simulink library "dspspect2"  (Simulink 3.00)
undefined symbols (not defined in the file or in its folder): magnitude
libraries: dspspect2 x5, dspparest2 x4, dspbdsp2 x2, dspxfrm2 x1, simulink x1, dsparch2 x1
settings Model: Creator=don  LastModifiedBy=surekha

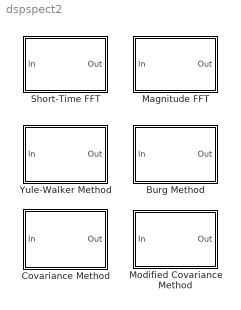
== system dspspect2 ==
  Burg Method : Subsystem  mask(Burg Method){fftsize=256, ord=6}
      mask prompts: fftsize "FFT length (-1 to inherit input width):"; ord "Order:"
      mask help: Frame-based parametric estimation of the AR spectrum using the Burg Method.
      mask init:
      | d = 0.1; xe=4; x=-xe:d:xe;
      | y = ones(size(x)); i=find(x); y(i)=sin(pi*x(i))./(pi*x(i));
      | y = abs(y).^(0.75);
      mask Help: web(dspbhelp);
      mask Display: text(-3,1.2,'Burg'); plot(-xe,0,xe,1.3,x,y)
  Covariance Method : Subsystem  mask(Covariance Method){bufsiz=128, fftsize=256, ord=6}
      mask prompts: bufsiz "Input frame size:"; fftsize "FFT length (-1 to inherit input width):"; ord "Order:"
      mask help: Frame-based parametric estimation of the AR spectrum using the Covariance Method.
      mask init:
      | d = 0.1; xe=4; x=-xe:d:xe;
      | y = ones(size(x)); i=find(x); y(i)=sin(pi*x(i))./(pi*x(i));
      | y = abs(y).^(0.75);
      mask Help: web(dspbhelp);
      mask Display: text(-3,1.2,'Cov AR'); plot(-xe,0,xe,1.3,x,y)
  Magnitude FFT : Subsystem  mask(Magnitude FFT){fftsize=128, NChans=1}
      mask prompts: fftsize "FFT length (-1 to inherit input width):"; NChans "Number of channels:"
      mask help: Compute magnitude-squared FFT of input frame, with optional zero padding.
      mask Help: web(dspbhelp);
      mask Display: disp('|FFT| ^ 2')
  Modified Covariance Method : Subsystem  mask(Modified Covariance Method){bufsiz=128, fftsize=256, ord=6}
      mask prompts: bufsiz "Input frame size:"; fftsize "FFT length (-1 to inherit input width):"; ord "Order:"
      mask help: Frame-based parametric estimation of the AR spectrum using the Modified Covariance Method.
      mask init:
      | d = 0.1; xe=4; x=-xe:d:xe;
      | y = ones(size(x)); i=find(x); y(i)=sin(pi*x(i))./(pi*x(i));
      | y = abs(y).^(0.75);
      mask Help: web(dspbhelp);
      mask Display: text(-3,1.2,'MCov AR'); plot(-xe,0,xe,1.3,x,y)
  Short-Time FFT : Subsystem  mask(Short-Time FFT){fftsize=256, navg=4, wintype=Hamming, Rs=50, beta=5, winsamp=Symmetric, NChans=1}
      mask prompts: fftsize "FFT length (-1 to inherit input width):"; navg "Number of spectral averages:"; wintype "Window type:"; Rs "Stopband attenuation in dB:"; winsamp "Window sampling:"; NChans "Number of channels:"
      mask help: Frame-based nonparametric spectral estimation using the short-time FFT.
      mask init:
      | [x,y,xe]=dspblkperiodogram('icon');
      mask Help: web(dspbhelp);
      mask StyleString: edit,edit,popup(Bartlett|Blackman|Boxcar|Chebyshev|Hamming|Hann|Hanning|Kaiser|Triang),edit,edit,popup(Symmetric|Periodic),edit
      mask CallbackString: ||dspblkperiodogram||||
      mask Display: text(-3,1.15,'ST-FFT'); plot(-xe,0,xe,1.3,x,y)
  Yule-Walker Method : Subsystem  mask(Yule-Walker Method){fftsize=256, ord=6}
      mask prompts: fftsize "FFT length (-1 to inherit input width):"; ord "Order:"
      mask help: Frame-based parametric estimation of the AR spectrum using the autocorrelation (LPC) method.
      mask init:
      | d = 0.1; xe=4; x=-xe:d:xe;
      | y = ones(size(x)); i=find(x); y(i)=sin(pi*x(i))./(pi*x(i));
      | y = abs(y).^(0.75);
      mask Help: web(dspbhelp);
      mask Display: text(-3,1.2,'Yule AR'); plot(-xe,0,xe,1.3,x,y)

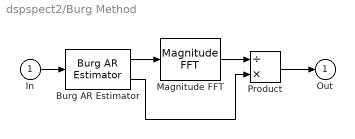
== system dspspect2/Burg Method ==
  In : Inport  Port=1  PortWidth=-1  SampleTime=-1  DataType=auto
      settings: SignalType=auto
  Burg AR Estimator : dspparest2/Burg AR Estimator  fcn=A  ord=ord
  Magnitude FFT : dspspect2/Magnitude FFT  fftsize=fftsize  NChans=1
  Product : Product  Inputs=/*  SaturateOnIntegerOverflow=on
  Out : Outport  Port=1  InitialOutput=0
  wires:
  In/1 -> Burg AR Estimator/1
  Burg AR Estimator/1 -> Magnitude FFT/1
  Magnitude FFT/1 -> Product/1
  Product/1 -> Out/1
  Burg AR Estimator/2 -> Product/2

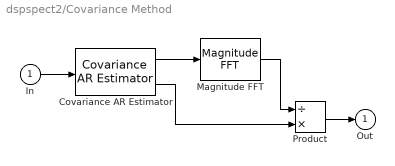
== system dspspect2/Covariance Method ==
  In : Inport  Port=1  PortWidth=-1  SampleTime=-1  DataType=auto
      settings: SignalType=auto
  Covariance AR Estimator : dspparest2/Covariance AR Estimator  bufsiz=bufsiz  ord=ord
  Magnitude FFT : dspspect2/Magnitude FFT  fftsize=fftsize  NChans=1
  Product : Product  Inputs=/*  SaturateOnIntegerOverflow=on
  Out : Outport  Port=1  InitialOutput=0
  wires:
  Magnitude FFT/1 -> Product/1
  Product/1 -> Out/1
  Covariance AR Estimator/1 -> Magnitude FFT/1
  Covariance AR Estimator/2 -> Product/2
  In/1 -> Covariance AR Estimator/1

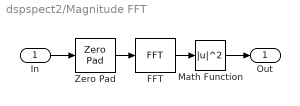
== system dspspect2/Magnitude FFT ==
  In : Inport  Port=1  PortWidth=-1  SampleTime=-1  DataType=auto
      settings: SignalType=auto
  FFT : dspxfrm2/FFT  nchans=NChans
  Math Function : Math  Operator=magnitude^2  OutputSignalType=auto
  Zero Pad : dspbdsp2/Zero Pad  pad=fftsize  trunc=on  nchans=NChans
  Out : Outport  Port=1
  wires:
  Math Function/1 -> Out/1
  In/1 -> Zero Pad/1
  Zero Pad/1 -> FFT/1
  FFT/1 -> Math Function/1

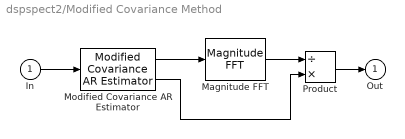
== system dspspect2/Modified Covariance Method ==
  In : Inport  Port=1  PortWidth=-1  SampleTime=-1  DataType=auto
      settings: SignalType=auto
  Magnitude FFT : dspspect2/Magnitude FFT  fftsize=fftsize  NChans=1
  Modified Covariance AR Estimator : dspparest2/Modified Covariance AR Estimator  bufsiz=bufsiz  ord=ord
  Product : Product  Inputs=/*  SaturateOnIntegerOverflow=on
  Out : Outport  Port=1  InitialOutput=0
  wires:
  In/1 -> Modified Covariance AR Estimator/1
  Modified Covariance AR Estimator/1 -> Magnitude FFT/1
  Magnitude FFT/1 -> Product/1
  Product/1 -> Out/1
  Modified Covariance AR Estimator/2 -> Product/2

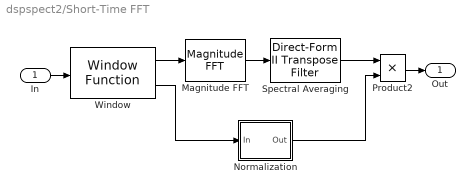
== system dspspect2/Short-Time FFT ==
  In : Inport  Port=1  PortWidth=-1  SampleTime=-1  DataType=auto
      settings: SignalType=auto
  Magnitude FFT : dspspect2/Magnitude FFT  fftsize=fftsize  NChans=NChans
  Normalization : Subsystem
  Product2 : Product  Inputs=**  SaturateOnIntegerOverflow=on
  Spectral Averaging : dsparch2/Direct-Form II Transpose Filter  num=ones(navg,1)/navg  den=1  ic=0  frame=off  numCHANS=1
  Window : dspbdsp2/Window Function  winmode=Generate and apply window  wintype=Hamming  N=64  Rs=Rs  beta=beta  winsamp=Symmetric  NChans=NChans
  Out : Outport  Port=1  InitialOutput=0
  wires:
  In/1 -> Window/1
  Magnitude FFT/1 -> Spectral Averaging/1
  Window/1 -> Magnitude FFT/1
  Product2/1 -> Out/1
  Spectral Averaging/1 -> Product2/1
  Normalization/1(Out) -> Product2/2
  Window/2 -> Normalization/1(In)

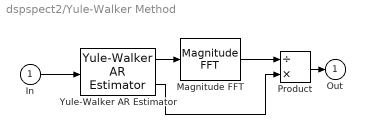
== system dspspect2/Yule-Walker Method ==
  In : Inport  Port=1  PortWidth=-1  SampleTime=-1  DataType=auto
      settings: SignalType=auto
  Magnitude FFT : dspspect2/Magnitude FFT  fftsize=fftsize  NChans=1
  Product : Product  Inputs=/*  SaturateOnIntegerOverflow=on
  Yule-Walker AR Estimator : dspparest2/Yule-Walker AR Estimator  ord=ord
  Out : Outport  Port=1  InitialOutput=0
  wires:
  Product/1 -> Out/1
  Yule-Walker AR Estimator/1 -> Magnitude FFT/1
  Magnitude FFT/1 -> Product/1
  Yule-Walker AR Estimator/2 -> Product/2
  In/1 -> Yule-Walker AR Estimator/1

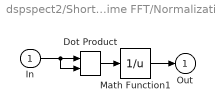
== system dspspect2/Short-Time FFT/Normalization ==
  In : Inport  Port=1  PortWidth=-1  SampleTime=-1  DataType=auto
      settings: SignalType=auto
  Dot Product : simulink/Linear/Dot Product
  Math Function1 : Math  Operator=reciprocal  OutputSignalType=auto
  Out : Outport  Port=1
  wires:
  Dot Product/1 -> Math Function1/1
  Math Function1/1 -> Out/1
  In/1 -> Dot Product/1, Dot Product/2
